simulink model "pmsm_sysid"  (R2021a)
settings: Solver=VariableStepAuto  StartTime=0.0  StopTime=6  RelTol=1e-3
model workspace (MATLAB code in the model file):
  | np=4; % pole pairs
  | phiv=0.1167; % rotor flux, wb
  | Kt=3/2*np*phiv;
  | f=7.43e-5; %Nm/(rad/s), friction
  | J=1.74e-4; %kgm*m, inertia
  | L=0.004; %H, inductance
  | Ld=L;
  | Lq=L;
  | Rs=1.74; %Ohm, armature resistance
  | Kp=50; % Prop gain in inner PI
  | Ki=2500; % I gain in inner PI
  | hh = 1e-2; % Sampling period
  | wN = pi/hh; % Nyquist freq
  | wBf = 0.7*wN; % Cutoff freq for AA filter
  | w0f = wBf/2.11; % AA filter param
values from neighbouring files (symbols this model uses):
  h = simres.uy.Time(3)- simres.uy.Time(2)    [pmsm_sysid_example.m]    (also in sysid_crane_example.m = 0.2; sysid_data.m = 1; sysid_data_hw_2019.m = 0.1; sysid_dc_fall18.m = 0.3)
settings Model: Creator=kjartan  LastModifiedBy=kjartan
settings SolverCC: AlgebraicLoopSolver=TrustRegion
settings DataIOCC: ReturnWorkspaceOutputs=off
settings DebuggingCC: SFMachineParentedDataDiag=warning  ArithmeticOperatorsInVariantConditions=warning
settings SFSimCC: CustomCodeUndefinedFunction=UseInterfaceOnly

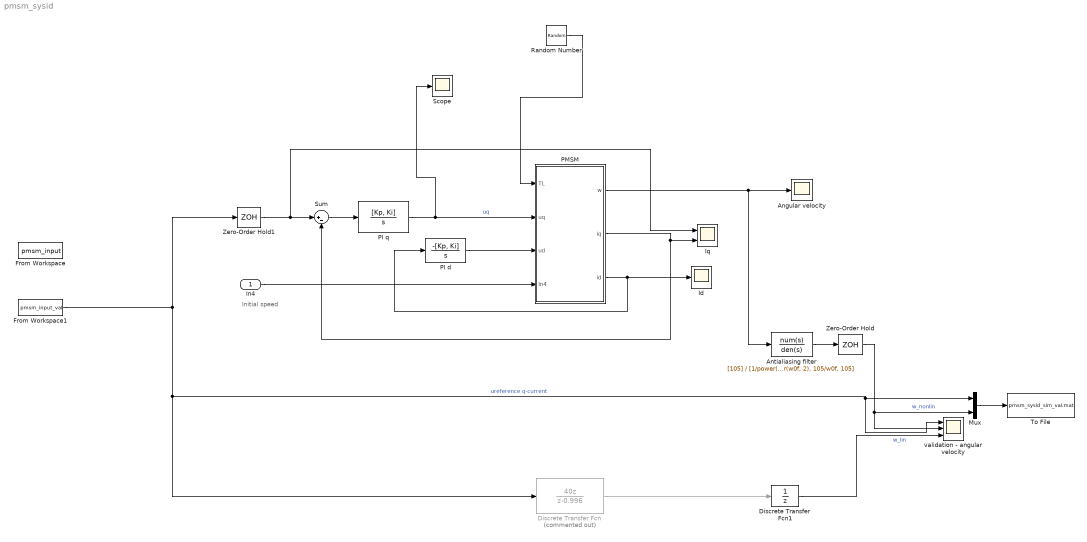
== system pmsm_sysid ==
  note: Initial speed
  In4 : Inport
  Angular velocity : Scope
  Antialiasing filter : TransferFcn  Numerator=[105]  Denominator=[1/power(w0f,4), 10/power(w0f, 3), 45/power(w0f, 2), 105/w0f, 105]
  Discrete Transfer Fcn : DiscreteTransferFcn  Commented=on  Numerator=[40, 0]  Denominator=[1 -0.996]  SampleTime=h
  Discrete Transfer Fcn1 : DiscreteTransferFcn  Denominator=[1 0]  SampleTime=h
  From Workspace : FromWorkspace  VariableName=pmsm_input  SampleTime=h
  From Workspace1 : FromWorkspace  VariableName=pmsm_input_val  SampleTime=h
  Id : Scope
  Iq : Scope  NumInputPorts=2
  Mux : Mux  Inputs=2
  PI d : TransferFcn  Numerator=-[Kp, Ki]  Denominator=[1, 0]
  PI q : TransferFcn  Numerator=[Kp, Ki]  Denominator=[1, 0]
  PMSM : Subsystem
  Random Number : RandomNumber  Variance=4  Seed=4  SampleTime=h
  Scope : Scope
  Sum : Sum  Inputs=|+-
  To File : ToFile  Filename=pmsm_sysid_sim_val.mat  MatrixName=uy  SaveFormat=Timeseries
  Zero-Order Hold : ZeroOrderHold  SampleTime=h
  Zero-Order Hold1 : ZeroOrderHold  SampleTime=h
  "validation - angular velocity " : Scope  NumInputPorts=3
  wires:
  PI q/1 -> Scope/1, PMSM/2(uq)  "uq"
  In4/1 -> PMSM/4(In4)
  PMSM/1(w) -> Angular velocity/1, Antialiasing filter/1
  PMSM/2(iq) -> Sum/2, Iq/2
  PMSM/3(id) -> PI d/1, Id/1
  Sum/1 -> PI q/1
  From Workspace1/1 -> Zero-Order Hold1/1, Mux/1, "validation - angular velocity "/1, Discrete Transfer Fcn/1  "ureference q-current"
  PI d/1 -> PMSM/3(ud)
  Zero-Order Hold1/1 -> Iq/1, Sum/1
  Antialiasing filter/1 -> Zero-Order Hold/1
  Zero-Order Hold/1 -> Mux/2, "validation - angular velocity "/2  "w_nonlin"
  Discrete Transfer Fcn/1 -> Discrete Transfer Fcn1/1
  Discrete Transfer Fcn1/1 -> "validation - angular velocity "/3  "w_lin"
  Mux/1 -> To File/1
  Random Number/1 -> PMSM/1(TL)

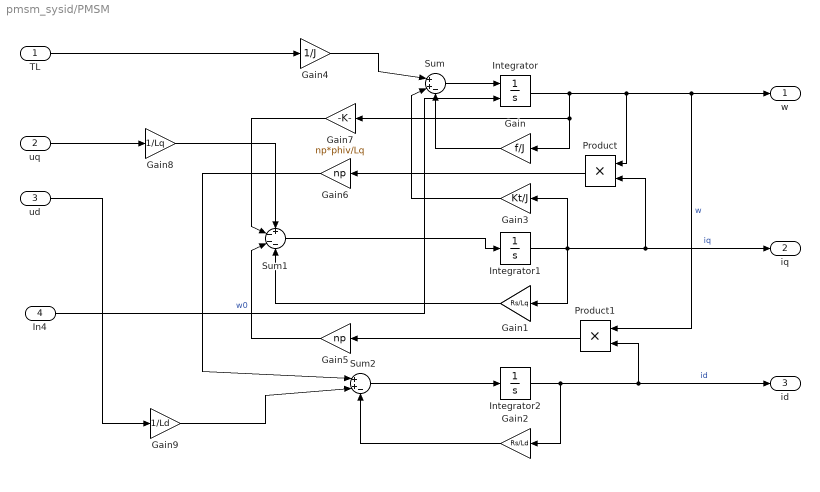
== system pmsm_sysid/PMSM ==
  TL : Inport
  uq : Inport  Port=2
  ud : Inport  Port=3
  In4 : Inport  Port=4
  Gain : Gain  Gain=f/J
  Gain1 : Gain  Gain=Rs/Lq
  Gain2 : Gain  Gain=Rs/Ld
  Gain3 : Gain  Gain=Kt/J
  Gain4 : Gain  Gain=1/J
  Gain5 : Gain  Gain=np
  Gain6 : Gain  Gain=np
  Gain7 : Gain  Gain=np*phiv/Lq
  Gain8 : Gain  Gain=1/Lq
  Gain9 : Gain  Gain=1/Ld
  Integrator : Integrator  InitialConditionSource=external
  Integrator1 : Integrator
  Integrator2 : Integrator
  Product : Product
  Product1 : Product
  Sum : Sum  Inputs=|++-
  Sum1 : Sum  Inputs=+---
  Sum2 : Sum  Inputs=|++-
  w : Outport  VectorParamsAs1DForOutWhenUnconnected=off
  iq : Outport  Port=2  VectorParamsAs1DForOutWhenUnconnected=off
  id : Outport  Port=3  VectorParamsAs1DForOutWhenUnconnected=off
  wires:
  Product/1 -> Gain6/1
  Gain9/1 -> Sum2/2
  Gain2/1 -> Sum2/3
  Gain5/1 -> Sum1/3
  Gain/1 -> Sum/3
  Gain8/1 -> Sum1/1
  Product1/1 -> Gain5/1
  Gain3/1 -> Sum/2
  Gain7/1 -> Sum1/2
  In4/1 -> Integrator/2  "w0"
  Integrator1/1 -> Gain3/1, Gain1/1, iq/1, Product/2  "iq"
  uq/1 -> Gain8/1
  Sum1/1 -> Integrator1/1
  Integrator/1 -> Gain7/1, Gain/1, Product/1, w/1, Product1/1  "w"
  Gain6/1 -> Sum2/1
  Sum2/1 -> Integrator2/1
  Gain1/1 -> Sum1/4
  Integrator2/1 -> Gain2/1, id/1, Product1/2  "id"
  ud/1 -> Gain9/1
  Sum/1 -> Integrator/1
  TL/1 -> Gain4/1
  Gain4/1 -> Sum/1
